simulink subsystem "Genset"  (R2022a)
settings: Solver=VariableStepAuto  StartTime=0.0  StopTime=10  RelTol=1e-3
model mask{Engine=Stellantis 3.0L, Generator=Yasa P400RHC x2}
  mask prompts: Engine "Select an Engine"; Generator "Select a Generator"
undefined symbols (not defined in the file or in its folder): Eng_BSFC_Map, Eng_Const_Power, Eng_Peak_RPM, Eng_Peak_Torque, Eng_RPM_Big, Eng_RPM_Map, Eng_Torque_Big, Eng_Torque_Map, Eng_Torque_Matrix, Gen_Max_Torque, Gen_Max_Torque_line, Gen_RPM_Map, Gen_Torque_Map, P_const_FCA, T_mat_FCA, w_CE_row
libraries: visionstatistics x4, simulink x2, slpidlib x1
settings Model: DefaultTestHarness=Genset_Harness3  Creator=kashyab  LastModifiedBy=kashyab

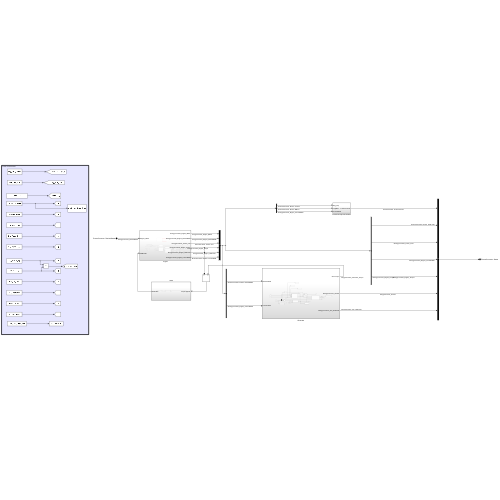
[thumbnail: Simulink's stored preview of the top-level diagram]
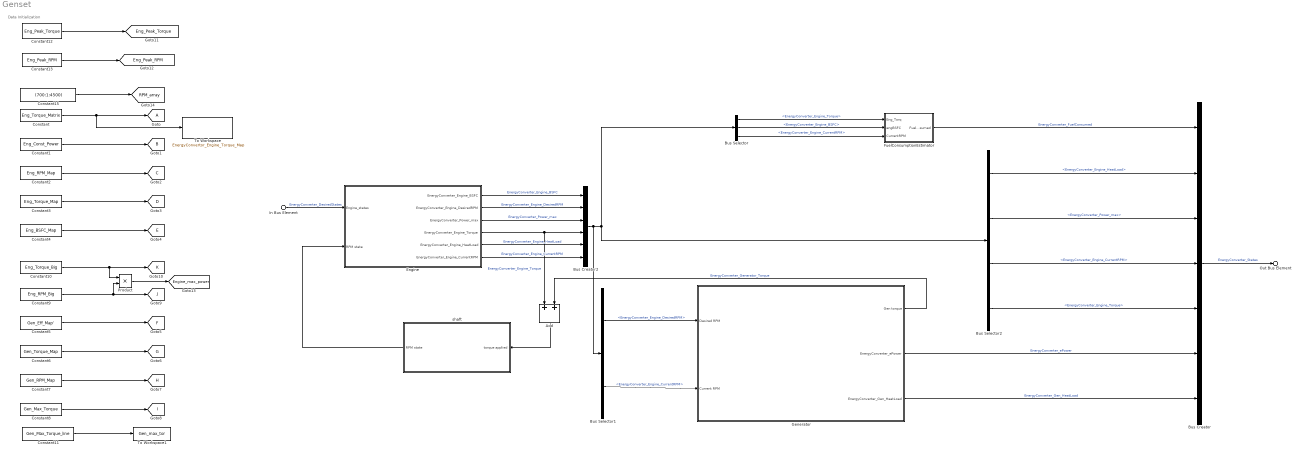
== system Genset ==
  note: Data Initialization
  In Bus Element : Inport  PortName=EnergyConverter_DesiredStates
  Add : Sum
  Bus Creator : BusCreator  Inputs=7
  Bus Creator2 : BusCreator  Inputs=6
  Bus Selector : BusSelector  OutputSignals=EnergyConverter_Engine_Torque,EnergyConverter_Engine_BSFC,EnergyConverter_Engine_CurrentRPM
  Bus Selector1 : BusSelector  OutputSignals=EnergyConverter_Engine_DesiredRPM,EnergyConverter_Engine_CurrentRPM
  Bus Selector2 : BusSelector  OutputSignals=EnergyConverter_Engine_HeatLoad,EnergyConverter_Power_max,EnergyConverter_Engine_CurrentRPM,EnergyConverter_Engine_Torque
  Constant : Constant  Value=Eng_Torque_Matrix
  Constant1 : Constant  Value=Eng_Const_Power
  Constant10 : Constant  Value=Eng_Torque_Big
  Constant11 : Constant  Value=Gen_Max_Torque_line
  Constant12 : Constant  Value=Eng_Peak_Torque
  Constant13 : Constant  Value=Eng_Peak_RPM
  Constant15 : Constant  Value=(700:1:4500)
  Constant2 : Constant  Value=Eng_RPM_Map
  Constant3 : Constant  Value=Eng_Torque_Map
  Constant4 : Constant  Value=Eng_BSFC_Map
  Constant5 : Constant  Value=Gen_Eff_Map'
  Constant6 : Constant  Value=Gen_Torque_Map
  Constant7 : Constant  Value=Gen_RPM_Map
  Constant8 : Constant  Value=Gen_Max_Torque
  Constant9 : Constant  Value=Eng_RPM_Big
  Engine : Subsystem
  FuelConsumptionEstimator : Subsystem
  Generator : Subsystem
  Goto : Goto  TagVisibility=global
  Product : Product
  To Workspace : ToWorkspace  VariableName=EnergyConvertor_Engine_Torque_Map  SampleTime=-1
      settings: Save2DSignal=2-D array (concatenate along first dimension)
  To Workspace1 : ToWorkspace  VariableName=Gen_max_tor  SaveFormat=Timeseries  SampleTime=-1
  shaft : Subsystem
  Out Bus Element : Outport  PortName=EnergyConverter_States
  tag scope: B=global, C=global, D=global, E=global, Eng_Peak_RPM=global, Eng_Peak_Torque=global, Engine_max_power=global, F=global, G=global, H=global, I=global, J=global, K=global, RPM_array=global
  wires:
  Generator/2(EnergyConverter_ePower) -> Bus Creator/6  "EnergyConverter_ePower"
  Bus Creator/1 -> Out Bus Element/1  "EnergyConverter_States"
  Constant8/1 -> [I]
  Constant7/1 -> [H]
  Constant6/1 -> [G]
  Constant5/1 -> [F]
  Constant4/1 -> [E]
  Constant3/1 -> [D]
  Constant2/1 -> [C]
  Constant1/1 -> [B]
  Constant/1 -> Goto/1, To Workspace/1
  Add/1 -> shaft/1("torque applied ")
  shaft/1(RPM state) -> Engine/2(RPM state)
  Generator/1("Gen torque ") -> Add/2  "EnergyConverter_Generator_Torque"
  Bus Selector2/3 -> Bus Creator/4  "<EnergyConverter_Engine_CurrentRPM>"
  Bus Selector2/2 -> Bus Creator/3  "<EnergyConverter_Power_max>"
  Constant9/1 -> [J], Product/2
  Generator/3(EnergyConverter_Gen_HeatLoad) -> Bus Creator/7  "EnergyConverter_Gen_HeatLoad"
  FuelConsumptionEstimator/1(FuelConsumed) -> Bus Creator/1  "EnergyConverter_FuelConsumed"
  Bus Selector2/1 -> Bus Creator/2  "<EnergyConverter_Engine_HeatLoad>"
  Constant11/1 -> To Workspace1/1
  Constant12/1 -> [Eng_Peak_Torque]
  Constant13/1 -> [Eng_Peak_RPM]
  Constant10/1 -> Product/1, [K]
  Product/1 -> [Engine_max_power]
  Constant15/1 -> [RPM_array]
  Engine/1(EnergyConverter_Engine_BSFC) -> Bus Creator2/1  "EnergyConverter_Engine_BSFC"
  Engine/2(EnergyConverter_Engine_DesiredRPM) -> Bus Creator2/2  "EnergyConverter_Engine_DesiredRPM"
  Engine/3(EnergyConverter_Power_max) -> Bus Creator2/3  "EnergyConverter_Power_max"
  Engine/4(" EnergyConverter_Engine_Torque") -> Bus Creator2/4, Add/1  "EnergyConverter_Engine_Torque"
  Engine/5(EnergyConverter_Engine_HeatLoad) -> Bus Creator2/5  "EnergyConverter_Engine_HeatLoad"
  Engine/6(EnergyConverter_Engine_CurrentRPM) -> Bus Creator2/6  "EnergyConverter_Engine_CurrentRPM"
  Bus Creator2/1 -> Bus Selector/1, Bus Selector2/1, Bus Selector1/1
  Bus Selector/1 -> FuelConsumptionEstimator/1(Eng_Torq)  "<EnergyConverter_Engine_Torque>"
  Bus Selector/2 -> FuelConsumptionEstimator/2(engBSFC)  "<EnergyConverter_Engine_BSFC>"
  Bus Selector/3 -> FuelConsumptionEstimator/3(CurrentRPM)  "<EnergyConverter_Engine_CurrentRPM>"
  Bus Selector1/1 -> Generator/1(Desired RPM)  "<EnergyConverter_Engine_DesiredRPM>"
  Bus Selector1/2 -> Generator/2(Current RPM)  "<EnergyConverter_Engine_CurrentRPM>"
  In Bus Element/1 -> Engine/1(Engine_states)  "EnergyConverter_DesiredStates"
  Bus Selector2/4 -> Bus Creator/5  "<EnergyConverter_Engine_Torque>"

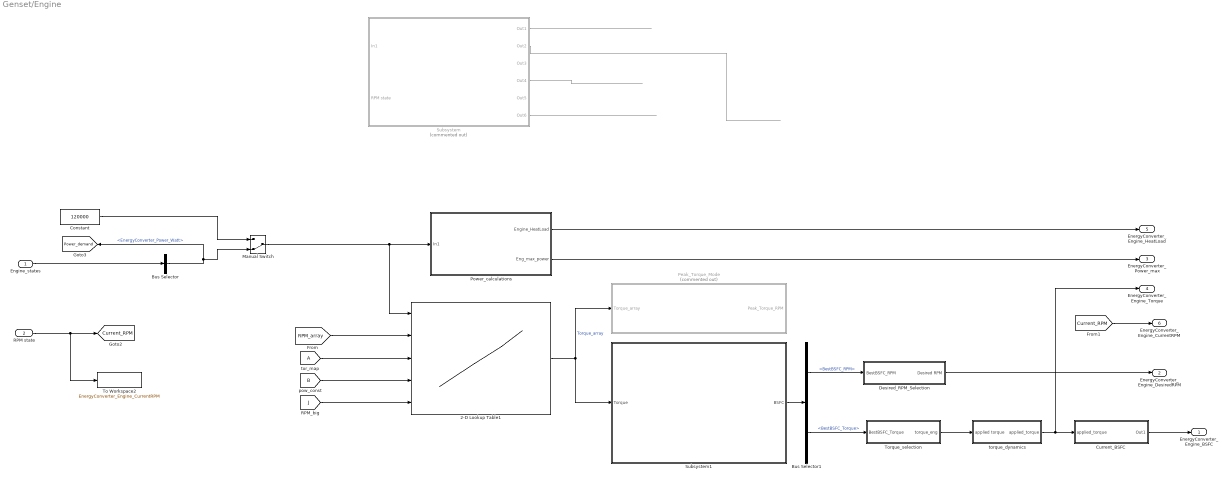
== system Genset/Engine ==
  Engine_states : Inport
  RPM state : Inport  Port=2
  2-D Lookup Table1 : Lookup_n-D  BreakpointsForDimension1Source=Input port  BreakpointsForDimension1=P_const_FCA  BreakpointsForDimension2Source=Input port  BreakpointsForDimension2=w_CE_row  IndexSearchMethod=Linear search  TableSource=Input port  Table=T_mat_FCA  ExtrapMethod=Clip  UseLastTableValue=on  InternalRulePriority=Speed  RndMeth=Simplest
      settings: InputPortMap=u0,u1,p221,p5,p7
  Bus Selector : BusSelector  OutputSignals=EnergyConverter_Power_Watt
  Bus Selector1 : BusSelector  OutputSignals=BestBSFC_RPM,BestBSFC_Torque
  Constant : Constant  Value=120000
  Current_BSFC : Subsystem
  Desired_RPM_Selection : Subsystem
  Manual Switch : ManualSwitch  CurrentSetting=0
  Peak_Torque_Mode : Subsystem  Commented=on
  Power_calculations : Subsystem
  Subsystem : Subsystem  Commented=on
  Subsystem1 : Subsystem
  To Workspace2 : ToWorkspace  VariableName=EnergyConverter_Engine_CurrentRPM  SampleTime=-1
      settings: Save2DSignal=2-D array (concatenate along first dimension)
  Torque_selection : Subsystem
  tor_map : From  TagVisibility=global
  torque_dynamics : Subsystem
  EnergyConverter_Engine_BSFC : Outport
  EnergyConverter_Engine_DesiredRPM : Outport  Port=2
  EnergyConverter_Power_max : Outport  Port=3
  " EnergyConverter_Engine_Torque" : Outport  Port=4
  EnergyConverter_Engine_HeatLoad : Outport  Port=5
  EnergyConverter_Engine_CurrentRPM : Outport  Port=6
  tag scope: Current_RPM=global, Power_demand=global
  wires:
  [RPM_array] -> 2-D Lookup Table1/2
  2-D Lookup Table1/1 -> Peak_Torque_Mode/1(Torque_array), Subsystem1/1(Torque)  "Torque_array"
  [B] -> 2-D Lookup Table1/4
  [J] -> 2-D Lookup Table1/5
  tor_map/1 -> 2-D Lookup Table1/3
  Subsystem/6(Out6) -> ?
  Subsystem/4(Out4) -> ?
  Subsystem/2(Out2) -> ?
  Subsystem/1(Out1) -> ?
  RPM state/1 -> [Current_RPM], To Workspace2/1
  Manual Switch/1 -> Power_calculations/1(In1), 2-D Lookup Table1/1
  Bus Selector/1 -> Manual Switch/2, [Power_demand]  "<EnergyConverter_Power_Watt>"
  Engine_states/1 -> Bus Selector/1
  Constant/1 -> Manual Switch/1
  Subsystem1/1(BSFC) -> Bus Selector1/1
  Bus Selector1/1 -> Desired_RPM_Selection/1(BestBSFC_RPM)  "<BestBSFC_RPM>"
  Bus Selector1/2 -> Torque_selection/1(BestBSFC_Torque)  "<BestBSFC_Torque>"
  Desired_RPM_Selection/1("Desired RPM ") -> EnergyConverter_Engine_DesiredRPM/1
  Torque_selection/1(torque_eng) -> torque_dynamics/1(applied torque)
  torque_dynamics/1(applied_torque) -> " EnergyConverter_Engine_Torque"/1, Current_BSFC/1(applied_torque)
  Current_BSFC/1(Out1) -> EnergyConverter_Engine_BSFC/1
  Power_calculations/2(Eng_max_power) -> EnergyConverter_Power_max/1
  Power_calculations/1(Engine_HeatLoad) -> EnergyConverter_Engine_HeatLoad/1
  [Current_RPM] -> EnergyConverter_Engine_CurrentRPM/1

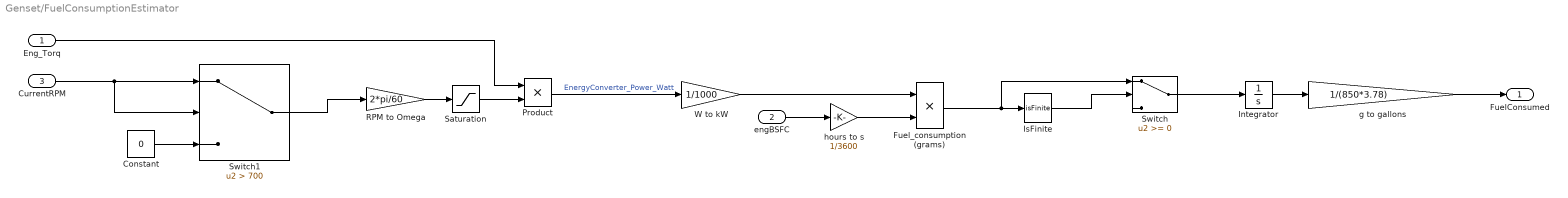
== system Genset/FuelConsumptionEstimator ==
  Eng_Torq : Inport
  engBSFC : Inport  Port=2
  CurrentRPM : Inport  Port=3
  Constant : Constant  Value=0
  Fuel_consumption (grams) : Product
  Integrator : Integrator
  IsFinite : RelationalOperator  Operator=isFinite  OutDataTypeStr=boolean  RndMeth=Simplest  InputSameDT=off
  Product : Product
  RPM to Omega : Gain  Gain=2*pi/60
  Saturation : Saturate  UpperLimit=Inf  LowerLimit=0
  Switch : Switch  SaturateOnIntegerOverflow=off  InputSameDT=off
  Switch1 : Switch  Criteria=u2 > Threshold  Threshold=700  SaturateOnIntegerOverflow=off  InputSameDT=off
  W to kW : Gain  Gain=1/1000
  g to gallons : Gain  Gain=1/(850*3.78)
  hours to s : Gain  Gain=1/3600
  FuelConsumed : Outport
  wires:
  Switch1/1 -> RPM to Omega/1
  Constant/1 -> Switch1/3
  Saturation/1 -> Product/2
  Switch/1 -> Integrator/1
  IsFinite/1 -> Switch/2
  Fuel_consumption (grams)/1 -> IsFinite/1, Switch/1
  Integrator/1 -> g to gallons/1
  engBSFC/1 -> hours to s/1
  Product/1 -> W to kW/1  "EnergyConverter_Power_Watt"
  RPM to Omega/1 -> Saturation/1
  CurrentRPM/1 -> Switch1/1, Switch1/2
  Eng_Torq/1 -> Product/1
  g to gallons/1 -> FuelConsumed/1
  hours to s/1 -> Fuel_consumption (grams)/2
  W to kW/1 -> Fuel_consumption (grams)/1

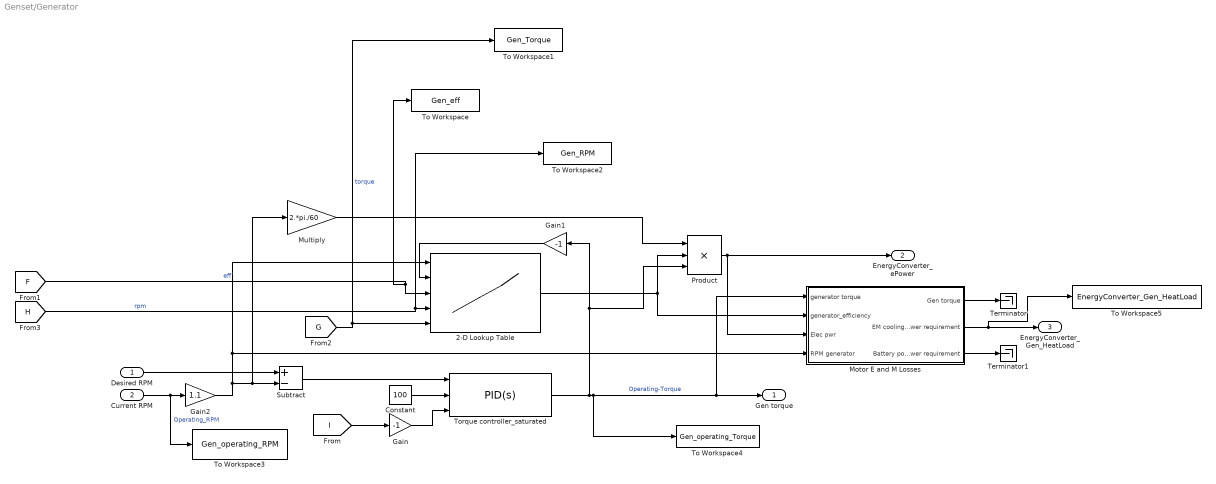
== system Genset/Generator ==
  Desired RPM : Inport
  Current RPM : Inport  Port=2
  2-D Lookup Table : Lookup_n-D  BreakpointsForDimension1Source=Input port  BreakpointsForDimension1=[1:3]  BreakpointsForDimension2Source=Input port  BreakpointsForDimension2=[1:3]  TableSource=Input port  ExtrapMethod=Clip  UseLastTableValue=on  InternalRulePriority=Speed  RndMeth=Simplest
      settings: InputPortMap=u0,u1,p221,p5,p7
  Constant : Constant  Value=100
  Gain : Gain  Gain=-1
  Gain1 : Gain  Gain=-1
  Gain2 : Gain  Gain=1.1
  Motor E and M Losses : Subsystem
  Multiply : Gain  Gain=2.*pi./60
  Product : Product  Inputs=3
  Subtract : Sum  Inputs=+-
  Terminator : Terminator
  Terminator1 : Terminator
  To Workspace : ToWorkspace  VariableName=Gen_eff  SaveFormat=Timeseries  SampleTime=-1
  To Workspace1 : ToWorkspace  VariableName=Gen_Torque  SaveFormat=Timeseries  SampleTime=-1
  To Workspace2 : ToWorkspace  VariableName=Gen_RPM  SaveFormat=Timeseries  SampleTime=-1
  To Workspace3 : ToWorkspace  VariableName=Gen_operating_RPM  SampleTime=-1
      settings: Save2DSignal=2-D array (concatenate along first dimension)
  To Workspace4 : ToWorkspace  VariableName=Gen_operating_Torque  SampleTime=-1
      settings: Save2DSignal=2-D array (concatenate along first dimension)
  To Workspace5 : ToWorkspace  VariableName=EnergyConverter_Gen_HeatLoad  SampleTime=-1
      settings: Save2DSignal=2-D array (concatenate along first dimension)
  Torque controller_saturated : slpidlib/PID Controller  Controller=PID  Form=Parallel  TimeDomain=Continuous-time  UseExternalTs=off  SampleTime=-1  IntegratorMethod=Forward Euler  FilterMethod=Forward Euler  ControllerParametersSource=internal  P=7.5  I=.5  UseKiTs=off  D=0  N=100  UseFilter=on  TunerSelectOption=Transfer Function Based (PID Tuner App)  InitialConditionSource=internal  InitialConditionForIntegrator=0  InitialConditionForFilter=0  DifferentiatorICPrevScaledInput=0  ExternalReset=none  TrackingMode=off  Kt=1  LimitOutput=on  SatLimitsSource=external  UpperSaturationLimit=0  LowerSaturationLimit=-650  LinearizeAsGain=on  AntiWindupMode=none  Kb=1  POutMin=[]  POutMax=[]  IOutMin=[]  IOutMax=[]  DOutMin=[]  DOutMax=[]  NOutMin=[]  NOutMax=[]  SumOutMin=[]  SumOutMax=[]  SaturationOutMin=[]  SaturationOutMax=[]  PParamMin=[]  PParamMax=[]  IParamMin=[]  IParamMax=[]  DParamMin=[]  DParamMax=[]  NParamMin=[]  NParamMax=[]  KbParamMin=[]  KbParamMax=[]  KtParamMin=[]  KtParamMax=[]  KbOutMin=[]  KbOutMax=[]  KtOutMin=[]  KtOutMax=[]  IntegratorOutMin=[]  IntegratorOutMax=[]  FilterOutMin=[]  FilterOutMax=[]  SumI1OutMin=[]  SumI1OutMax=[]  SumI2OutMin=[]  SumI2OutMax=[]  SumI3OutMin=[]  SumI3OutMax=[]  SumI4OutMin=[]  SumI4OutMax=[]  SumDOutMin=[]  SumDOutMax=[]  DifferentiatorOutMin=[]  DifferentiatorOutMax=[]  FilterDiffOutCoefMin=[]  FilterDiffOutCoefMax=[]  ReciprocalOutMin=[]  ReciprocalOutMax=[]  SumDenOutMin=[]  SumDenOutMax=[]  SumNumOutMin=[]  SumNumOutMax=[]  DivideOutMin=[]  DivideOutMax=[]  UdiffTsProdOutMin=[]  UdiffTsProdOutMax=[]  NTsProdOutMin=[]  NTsProdOutMax=[]  UintegralTsProdOutMin=[]  UintegralTsProdOutMax=[]  UngainTsProdOutMin=[]  UngainTsProdOutMax=[]  IntegratorContinuousStateAttributes=''  IntegratorStateMustResolveToSignalObject=off  IntegratorRTWStateStorageClass=Auto  FilterContinuousStateAttributes=''  FilterStateMustResolveToSignalObject=off  FilterRTWStateStorageClass=Auto  ParallelPVariant=InternalParameters  IdealPVariant=Disabled  IVariant=InternalParameters  DVariant=InternalParameters  IntegratorVariant=Continuous  SatVariant=External  AWVariant=Passthrough  PCopyVariant=Disabled  TRVariant=Disabled  FdbkBlocksVariant=Forward  IdealPFdbkVariant=Disabled  SatFdbkVariant=Disabled  DerivativeFilterVariant=ContFilter  NVariant=InternalParameters  NCopyVariant=Disabled  FilterICVariant=InternalICsFilter  IntegratorICVariant=InternalICs  ExternalResetVariant=Disabled  TRSumVariant=Passthrough  SumFdbkVariant=Disabled  SumVariant=Sum_PID  TsampFilterVariant=InternalTs  TsampNgainVariant=Passthrough  TsampIntegralVariant=Passthrough  ExternalSaturationOutDataTypeStr=Inherit: Same as second input  aMode=0
  "Gen torque " : Outport
  EnergyConverter_ePower : Outport  Port=2
  EnergyConverter_Gen_HeatLoad : Outport  Port=3
  wires:
  Gain2/1 -> 2-D Lookup Table/1, Motor E and M Losses/4(RPM generator), Multiply/1, Subtract/2
  Desired RPM/1 -> Subtract/1
  [F] -> 2-D Lookup Table/3, To Workspace/1  "eff"
  Torque controller_saturated/1 -> Motor E and M Losses/1(generator torque), "Gen torque "/1, To Workspace4/1, Gain1/1, Product/3  "Operating-Torque"
  Subtract/1 -> Torque controller_saturated/1
  Current RPM/1 -> To Workspace3/1, Gain2/1  "Operating_RPM"
  2-D Lookup Table/1 -> Product/2, Motor E and M Losses/2(generator_efficiency)
  Constant/1 -> Torque controller_saturated/2
  [I] -> Gain/1
  Gain/1 -> Torque controller_saturated/3
  Multiply/1 -> Product/1
  Product/1 -> Motor E and M Losses/3(Elec pwr), EnergyConverter_ePower/1
  [H] -> To Workspace2/1, 2-D Lookup Table/4  "rpm"
  [G] -> 2-D Lookup Table/5, To Workspace1/1  "torque"
  Gain1/1 -> 2-D Lookup Table/2
  Motor E and M Losses/3(Battery power requirement) -> Terminator1/1
  Motor E and M Losses/1(Gen torque) -> Terminator/1
  Motor E and M Losses/2(EM cooling power requirement) -> To Workspace5/1, EnergyConverter_Gen_HeatLoad/1

== system Genset/shaft ==
  "torque applied " : Inport
  Gain : Gain  Gain=10
  Integrator : Integrator  InitialCondition=1
  RPM state : Outport
  wires:
  Gain/1 -> Integrator/1
  Integrator/1 -> RPM state/1
  "torque applied "/1 -> Gain/1

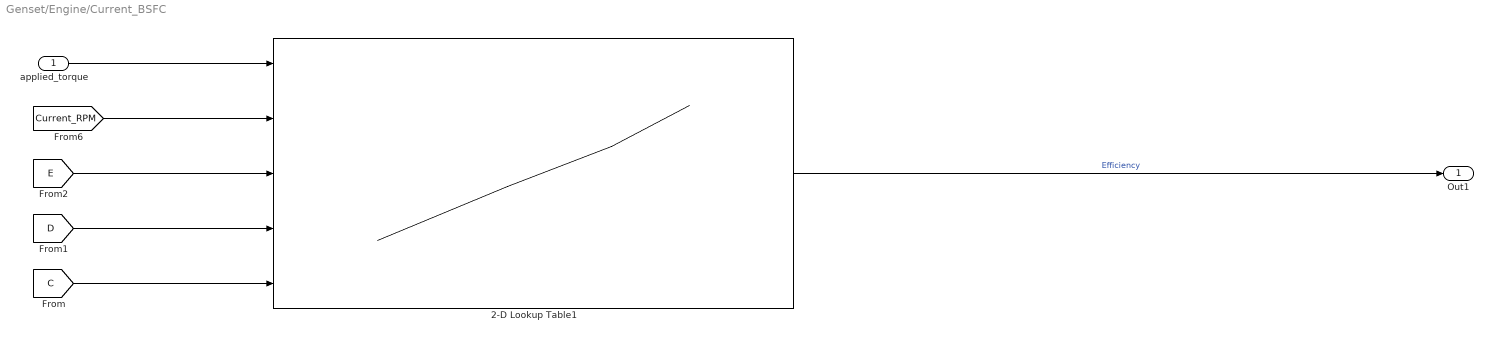
== system Genset/Engine/Current_BSFC ==
  applied_torque : Inport
  2-D Lookup Table1 : Lookup_n-D  BreakpointsForDimension1Source=Input port  BreakpointsForDimension1=[1:3]  BreakpointsForDimension2Source=Input port  BreakpointsForDimension2=[1:3]  TableSource=Input port  ExtrapMethod=Clip  UseLastTableValue=on  InternalRulePriority=Speed  RndMeth=Simplest
      settings: InputPortMap=u0,u1,p221,p5,p7
  Out1 : Outport
  wires:
  [Current_RPM] -> 2-D Lookup Table1/2
  2-D Lookup Table1/1 -> Out1/1  "Efficiency"
  applied_torque/1 -> 2-D Lookup Table1/1
  [D] -> 2-D Lookup Table1/4
  [E] -> 2-D Lookup Table1/3
  [C] -> 2-D Lookup Table1/5

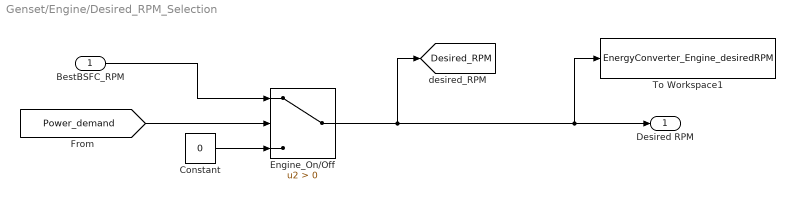
== system Genset/Engine/Desired_RPM_Selection ==
  BestBSFC_RPM : Inport
  Constant : Constant  Value=0
  Engine_On/Off : Switch  Criteria=u2 > Threshold  SaturateOnIntegerOverflow=off  InputSameDT=off
  To Workspace1 : ToWorkspace  VariableName=EnergyConverter_Engine_desiredRPM  SampleTime=-1
      settings: Save2DSignal=2-D array (concatenate along first dimension)
  "Desired RPM " : Outport
  tag scope: Desired_RPM=global
  wires:
  Engine_On/Off/1 -> "Desired RPM "/1, To Workspace1/1, [Desired_RPM]
  [Power_demand] -> Engine_On/Off/2
  Constant/1 -> Engine_On/Off/3
  BestBSFC_RPM/1 -> Engine_On/Off/1

== system Genset/Engine/Peak_Torque_Mode ==
  Torque_array : Inport
  Max RPM : MultiPortSwitch  DataPortOrder=Zero-based contiguous  Inputs=1  zeroidx=on  SaturateOnIntegerOverflow=off  InputSameDT=off
  Max Torque : visionstatistics/2-D Maximum  fcn=Index  reset=None  indexBase=One  operateOver=Entire input  Dimension=1  colComp=on  operation=maximum  accumLastDataTypeStr=Inherit: Same as product output  roiEnable=off  roiType=Rectangles  roiPortion=Entire ROI  roiOutput=Individual statistics for each ROI  roiFlag=off  roundingMode=Floor  overflowMode=off  accumDataTypeStr=Inherit: Same as product output
      settings: SourceProductBaseCode=VP
  Peak_Torque_RPM : Outport
  wires:
  Torque_array/1 -> Max Torque/1
  [RPM_array] -> Max RPM/2
  Max Torque/1 -> Max RPM/1
  Max RPM/1 -> Peak_Torque_RPM/1

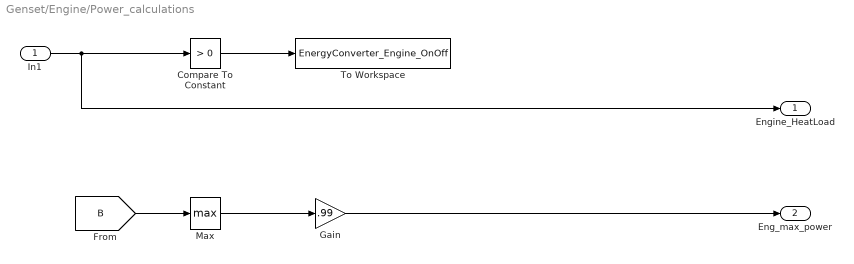
== system Genset/Engine/Power_calculations ==
  In1 : Inport
  Compare To Constant : simulink/Logic and Bit Operations/Compare To Constant  relop=>  const=0  OutDataTypeStr=boolean
  Gain : Gain  Gain=.99
  Max : MinMax  Function=max
  To Workspace : ToWorkspace  VariableName=EnergyConverter_Engine_OnOff  SampleTime=-1
      settings: Save2DSignal=2-D array (concatenate along first dimension)
  Engine_HeatLoad : Outport
  Eng_max_power : Outport  Port=2
  wires:
  In1/1 -> Engine_HeatLoad/1, Compare To Constant/1
  Compare To Constant/1 -> To Workspace/1
  [B] -> Max/1
  Max/1 -> Gain/1
  Gain/1 -> Eng_max_power/1

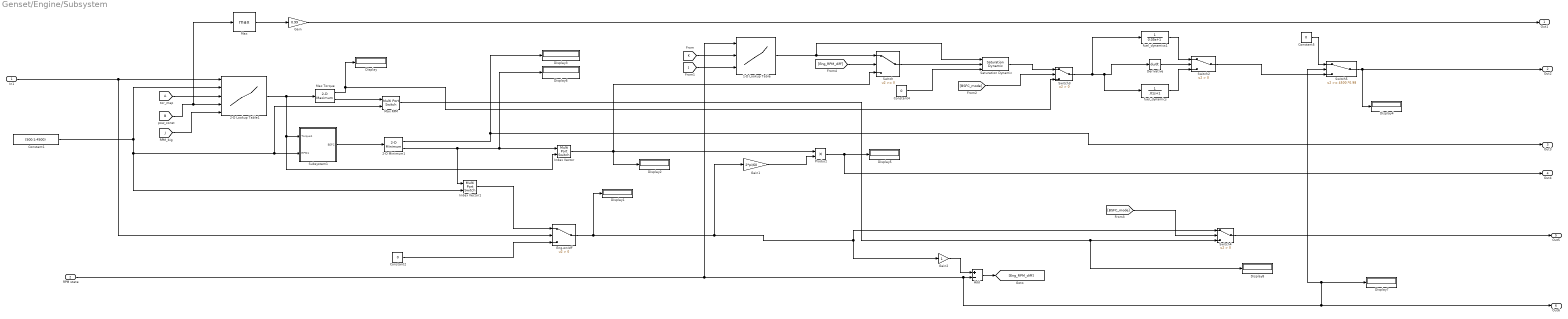
== system Genset/Engine/Subsystem ==
  In1 : Inport
  RPM state : Inport  Port=2
  1-D Lookup Table : Lookup_n-D  NumberOfTableDimensions=1  BreakpointsForDimension1Source=Input port  BreakpointsForDimension1=[-5:5]  TableSource=Input port  Table=tanh([-5:5])  ExtrapMethod=Clip  UseLastTableValue=on  InternalRulePriority=Speed  RndMeth=Simplest
      settings: InputPortMap=u0,p221,p5
  2-D Lookup Table1 : Lookup_n-D  BreakpointsForDimension1Source=Input port  BreakpointsForDimension1=P_const_FCA  BreakpointsForDimension2Source=Input port  BreakpointsForDimension2=w_CE_row  IndexSearchMethod=Linear search  TableSource=Input port  Table=T_mat_FCA  ExtrapMethod=Clip  UseLastTableValue=on  InternalRulePriority=Speed  RndMeth=Simplest
      settings: InputPortMap=u0,u1,p221,p5,p7
  2-D Minimum1 : visionstatistics/2-D Minimum  fcn=Value and Index  reset=None  indexBase=One  operateOver=Entire input  Dimension=1  colComp=on  operation=minimum  accumLastDataTypeStr=Inherit: Same as product output  roiEnable=off  roiType=Rectangles  roiPortion=Entire ROI  roiOutput=Individual statistics for each ROI  roiFlag=off  roundingMode=Floor  overflowMode=off  accumDataTypeStr=Inherit: Same as product output
      settings: SourceProductBaseCode=VP
  Add : Sum  Inputs=+-
  Constant1 : Constant  Value=(500:1:4500)
  Constant2 : Constant  Value=0
  Constant4 : Constant  Value=0
  Constant5 : Constant  Value=0
  Derivative : Derivative
  Display{,1..8} (9 alike) : Display
      Display3 settings: Decimation=4
      Display6 settings: Decimation=4
  Eng-on/off : Switch  Criteria=u2 > Threshold  SaturateOnIntegerOverflow=off  InputSameDT=off
  Gain : Gain  Gain=0.99
  Gain1 : Gain  Gain=2*pi/60
  Gain2 : Gain
  Index Vector : MultiPortSwitch  Inputs=1  SaturateOnIntegerOverflow=off  InputSameDT=off
  Index Vector1 : MultiPortSwitch  Inputs=1  SaturateOnIntegerOverflow=off  InputSameDT=off
  Max : MinMax  Function=max
  Max RPM : MultiPortSwitch  DataPortOrder=Zero-based contiguous  Inputs=1  zeroidx=on  SaturateOnIntegerOverflow=off  InputSameDT=off
  Max Torque : visionstatistics/2-D Maximum  fcn=Value and Index  reset=None  indexBase=One  operateOver=Entire input  Dimension=1  colComp=on  operation=maximum  accumLastDataTypeStr=Inherit: Same as product output  roiEnable=off  roiType=Rectangles  roiPortion=Entire ROI  roiOutput=Individual statistics for each ROI  roiFlag=off  roundingMode=Floor  overflowMode=off  accumDataTypeStr=Inherit: Same as product output
      settings: SourceProductBaseCode=VP
  Product : Product
  Saturation Dynamic : simulink/Discontinuities/Saturation Dynamic  OutMin=[]  OutMax=[]  OutDataTypeStr=Inherit: Same as second input  OutDataType=fixdt(1, 16)  OutScaling=2^-10  DoSatur=off
  Subsystem1 : Subsystem
  Switch : Switch  SaturateOnIntegerOverflow=off  InputSameDT=off
  Switch2 : Switch  Criteria=u2 > Threshold  SaturateOnIntegerOverflow=off  InputSameDT=off
  Switch3 : Switch  Criteria=u2 > Threshold  SaturateOnIntegerOverflow=off  InputSameDT=off
  Switch4 : Switch  Criteria=u2 > Threshold  SaturateOnIntegerOverflow=off  InputSameDT=off
  Switch5 : Switch  Threshold=4500.*0.98  SaturateOnIntegerOverflow=off  InputSameDT=off
  fuel_dynamics : TransferFcn  Denominator=[.01 1]
  fuel_dynamics1 : TransferFcn  Denominator=[0.05 1]
  tor_map : From  TagVisibility=global
  Out1 : Outport
  Out2 : Outport  Port=2
  Out3 : Outport  Port=3
  Out4 : Outport  Port=4
  Out5 : Outport  Port=5
  Out6 : Outport  Port=6
  wires:
  fuel_dynamics/1 -> Switch2/3
  fuel_dynamics1/1 -> Switch2/1
  Derivative/1 -> Switch2/2
  Switch3/1 -> Derivative/1, fuel_dynamics/1, fuel_dynamics1/1
  Constant4/1 -> Saturation Dynamic/3
  Max Torque/1 -> Switch3/3, Display/1
  In1/1 -> 2-D Lookup Table1/1, Eng-on/off/2
  1-D Lookup Table/1 -> Switch/1, Saturation Dynamic/1
  Add/1 -> [Eng_RPM_diff]
  Max/1 -> Gain/1
  tor_map/1 -> 2-D Lookup Table1/3
  RPM state/1 -> 1-D Lookup Table/1, Add/2, Switch5/2, Display7/1, Out6/1
  Switch4/1 -> Out5/1
  Gain/1 -> Out1/1
  [Eng_RPM_diff] -> Switch/2
  [J] -> 2-D Lookup Table1/5
  Max Torque/2 -> Max RPM/1
  [K] -> 1-D Lookup Table/2
  Gain2/1 -> Add/1
  Constant2/1 -> Eng-on/off/3
  Constant1/1 -> 2-D Lookup Table1/2, Index Vector1/2, Subsystem1/2(RPM1), Max RPM/2
  Index Vector/1 -> Switch/3, Display2/1, Product/1
  [BSFC_mode] -> Switch4/2
  Max RPM/1 -> Switch4/3, Display8/1
  2-D Lookup Table1/1 -> Index Vector/2, Subsystem1/1(Torque1), Max Torque/1
  Saturation Dynamic/1 -> Switch3/1
  [J] -> 1-D Lookup Table/3
  [BSFC_mode] -> Switch3/2
  Index Vector1/1 -> Eng-on/off/1
  2-D Minimum1/2 -> Display6/1, Index Vector/1, Index Vector1/1
  Subsystem1/1(BSFC) -> 2-D Minimum1/1
  Switch5/1 -> Display4/1, Out2/1
  Switch2/1 -> Switch5/3
  Constant5/1 -> Switch5/1
  2-D Minimum1/1 -> Display3/1, Out3/1
  Product/1 -> Display5/1, Out4/1
  [B] -> Max/1, 2-D Lookup Table1/4
  Switch/1 -> Saturation Dynamic/2
  Eng-on/off/1 -> Display1/1, Gain1/1, Gain2/1, Switch4/1
  Gain1/1 -> Product/2

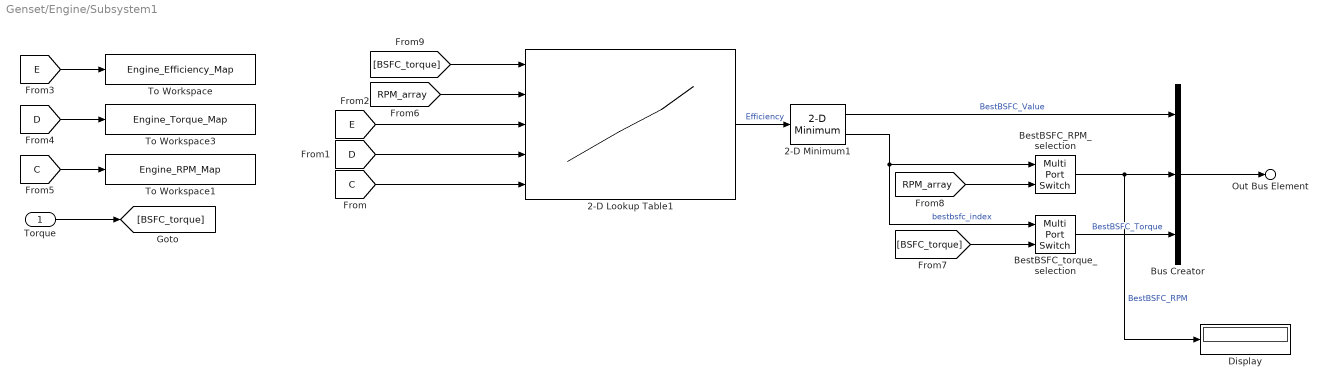
== system Genset/Engine/Subsystem1 ==
  Torque : Inport
  2-D Lookup Table1 : Lookup_n-D  BreakpointsForDimension1Source=Input port  BreakpointsForDimension1=[1:3]  BreakpointsForDimension2Source=Input port  BreakpointsForDimension2=[1:3]  TableSource=Input port  ExtrapMethod=Clip  UseLastTableValue=on  InternalRulePriority=Speed  RndMeth=Simplest
      settings: InputPortMap=u0,u1,p221,p5,p7
  2-D Minimum1 : visionstatistics/2-D Minimum  fcn=Value and Index  reset=None  indexBase=One  operateOver=Entire input  Dimension=1  colComp=on  operation=minimum  accumLastDataTypeStr=Inherit: Same as product output  roiEnable=off  roiType=Rectangles  roiPortion=Entire ROI  roiOutput=Individual statistics for each ROI  roiFlag=off  roundingMode=Floor  overflowMode=off  accumDataTypeStr=Inherit: Same as product output
      settings: SourceProductBaseCode=VP
  BestBSFC_RPM_selection : MultiPortSwitch  Inputs=1  SaturateOnIntegerOverflow=off  InputSameDT=off
  BestBSFC_torque_selection : MultiPortSwitch  Inputs=1  SaturateOnIntegerOverflow=off  InputSameDT=off
  Bus Creator : BusCreator  Inputs=3
  Display : Display
  To Workspace : ToWorkspace  VariableName=Engine_Efficiency_Map  SampleTime=-1
      settings: Save2DSignal=2-D array (concatenate along first dimension)
  To Workspace1 : ToWorkspace  VariableName=Engine_RPM_Map  SampleTime=-1
      settings: Save2DSignal=2-D array (concatenate along first dimension)
  To Workspace3 : ToWorkspace  VariableName=Engine_Torque_Map  SampleTime=-1
      settings: Save2DSignal=2-D array (concatenate along first dimension)
  Out Bus Element : Outport  PortName=BSFC
  wires:
  [BSFC_torque] -> 2-D Lookup Table1/1
  BestBSFC_torque_selection/1 -> Bus Creator/3  "BestBSFC_Torque"
  BestBSFC_RPM_selection/1 -> Bus Creator/2, Display/1  "BestBSFC_RPM"
  [RPM_array] -> BestBSFC_RPM_selection/2
  [BSFC_torque] -> BestBSFC_torque_selection/2
  Bus Creator/1 -> Out Bus Element/1
  2-D Minimum1/2 -> BestBSFC_RPM_selection/1, BestBSFC_torque_selection/1  "bestbsfc_index"
  2-D Minimum1/1 -> Bus Creator/1  "BestBSFC_Value"
  [C] -> To Workspace1/1
  [D] -> To Workspace3/1
  [E] -> To Workspace/1
  [C] -> 2-D Lookup Table1/5
  [RPM_array] -> 2-D Lookup Table1/2
  Torque/1 -> [BSFC_torque]
  2-D Lookup Table1/1 -> 2-D Minimum1/1  "Efficiency"
  [E] -> 2-D Lookup Table1/3
  [D] -> 2-D Lookup Table1/4

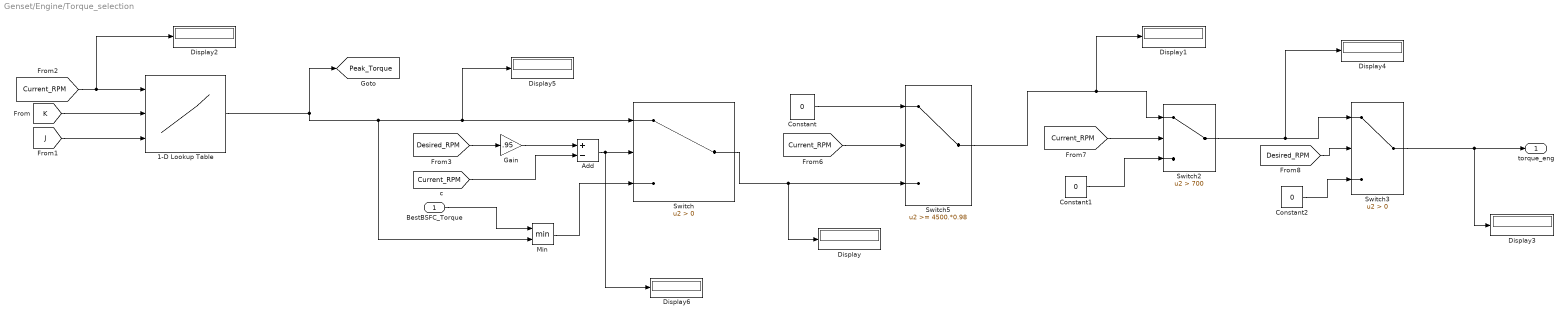
== system Genset/Engine/Torque_selection ==
  BestBSFC_Torque : Inport
  1-D Lookup Table : Lookup_n-D  NumberOfTableDimensions=1  BreakpointsForDimension1Source=Input port  BreakpointsForDimension1=[-5:5]  TableSource=Input port  Table=tanh([-5:5])  ExtrapMethod=Clip  UseLastTableValue=on  InternalRulePriority=Speed  RndMeth=Simplest
      settings: InputPortMap=u0,p221,p5
  Add : Sum  Inputs=+-
  Constant : Constant  Value=0
  Constant1 : Constant  Value=0
  Constant2 : Constant  Value=0
  Display{,1..6} (7 alike) : Display
  Gain : Gain  Gain=.95
  Min : MinMax  Inputs=2
  Switch : Switch  Criteria=u2 > Threshold  SaturateOnIntegerOverflow=off  InputSameDT=off
  Switch2 : Switch  Criteria=u2 > Threshold  Threshold=700  SaturateOnIntegerOverflow=off  InputSameDT=off
  Switch3 : Switch  Criteria=u2 > Threshold  SaturateOnIntegerOverflow=off  InputSameDT=off
  Switch5 : Switch  Threshold=4500.*0.98  SaturateOnIntegerOverflow=off  InputSameDT=off
  torque_eng : Outport
  tag scope: Peak_Torque=global
  wires:
  Min/1 -> Switch/3
  BestBSFC_Torque/1 -> Min/1
  Constant2/1 -> Switch3/3
  Switch3/1 -> torque_eng/1, Display3/1
  [Desired_RPM] -> Switch3/2
  Switch2/1 -> Switch3/1, Display4/1
  Switch5/1 -> Switch2/1, Display1/1
  Constant1/1 -> Switch2/3
  [Current_RPM] -> Switch2/2
  1-D Lookup Table/1 -> [Peak_Torque], Display5/1, Switch/1, Min/2
  [J] -> 1-D Lookup Table/3
  [Current_RPM] -> 1-D Lookup Table/1, Display2/1
  [K] -> 1-D Lookup Table/2
  [Desired_RPM] -> Gain/1
  [Current_RPM] -> Add/2
  Gain/1 -> Add/1
  Add/1 -> Switch/2, Display6/1
  [Current_RPM] -> Switch5/2
  Constant/1 -> Switch5/1
  Switch/1 -> Switch5/3, Display/1

== system Genset/Engine/torque_dynamics ==
  applied torque : Inport
  Derivative : Derivative
  Switch2 : Switch  Criteria=u2 > Threshold  SaturateOnIntegerOverflow=off  InputSameDT=off
  fuel_dynamics : TransferFcn  Denominator=[.01 1]
  fuel_dynamics1 : TransferFcn  Denominator=[0.05 1]
  applied_torque : Outport
  wires:
  Switch2/1 -> applied_torque/1
  applied torque/1 -> Derivative/1, fuel_dynamics/1, fuel_dynamics1/1
  fuel_dynamics1/1 -> Switch2/1
  fuel_dynamics/1 -> Switch2/3
  Derivative/1 -> Switch2/2

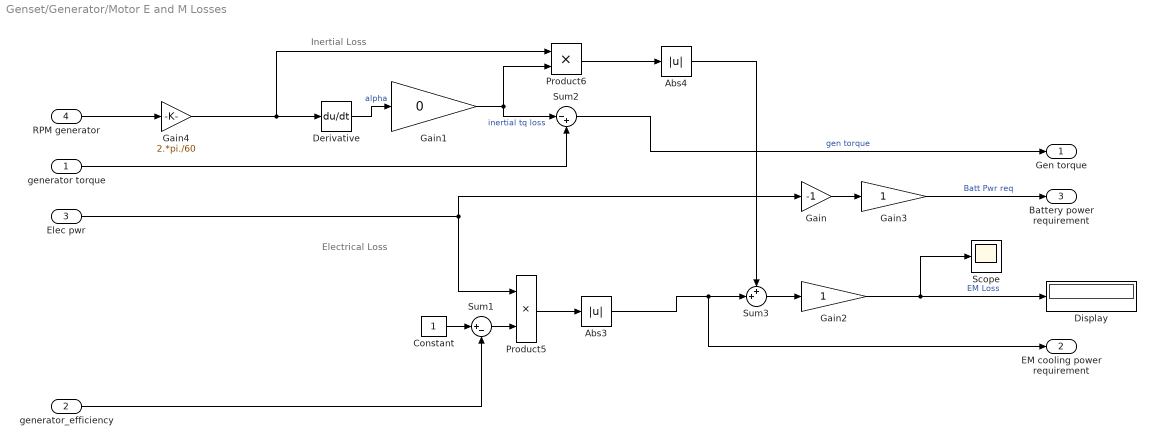
== system Genset/Generator/Motor E and M Losses ==
  note: Inertial Loss
  note: Electrical Loss
  generator torque : Inport
  generator_efficiency : Inport  Port=2
  Elec pwr : Inport  Port=3
  RPM generator : Inport  Port=4
  Abs3 : Abs  SaturateOnIntegerOverflow=off
  Abs4 : Abs  ZeroCross=off  SaturateOnIntegerOverflow=off
  Constant : Constant
  Derivative : Derivative
  Display : Display
  Gain : Gain  Gain=-1
  Gain1 : Gain  Gain=0
  Gain2 : Gain
  Gain3 : Gain
  Gain4 : Gain  Gain=2.*pi./60
  Product5 : Product
  Product6 : Product
  Scope : Scope
  Sum1 : Sum  Inputs=|+-
  Sum2 : Sum  Inputs=|-+
  Sum3 : Sum  Inputs=++|
  Gen torque : Outport
  EM cooling power requirement : Outport  Port=2
  Battery power requirement : Outport  Port=3
  wires:
  Gain4/1 -> Derivative/1, Product6/1
  Gain3/1 -> Battery power requirement/1  "Batt Pwr req"
  Gain/1 -> Gain3/1
  generator_efficiency/1 -> Sum1/2
  Sum2/1 -> Gen torque/1  "gen torque"
  Derivative/1 -> Gain1/1  "alpha"
  Elec pwr/1 -> Product5/1, Gain/1
  Product6/1 -> Abs4/1
  Constant/1 -> Sum1/1
  Abs4/1 -> Sum3/1
  Gain1/1 -> Sum2/1, Product6/2  "inertial tq loss"
  Product5/1 -> Abs3/1
  Gain2/1 -> Scope/1, Display/1  "EM Loss"
  Sum1/1 -> Product5/2
  Sum3/1 -> Gain2/1
  Abs3/1 -> Sum3/2, EM cooling power requirement/1
  RPM generator/1 -> Gain4/1
  generator torque/1 -> Sum2/2

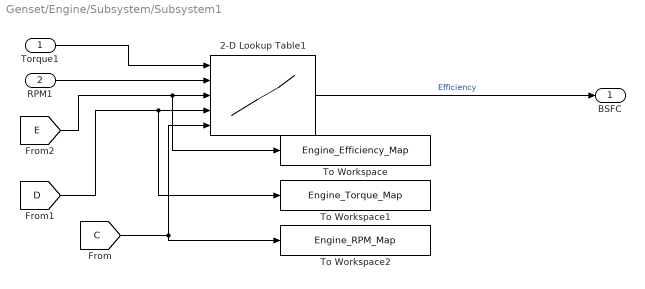
== system Genset/Engine/Subsystem/Subsystem1 ==
  Torque1 : Inport
  RPM1 : Inport  Port=2
  2-D Lookup Table1 : Lookup_n-D  BreakpointsForDimension1Source=Input port  BreakpointsForDimension1=[1:3]  BreakpointsForDimension2Source=Input port  BreakpointsForDimension2=[1:3]  TableSource=Input port  ExtrapMethod=Clip  UseLastTableValue=on  InternalRulePriority=Speed  RndMeth=Simplest
      settings: InputPortMap=u0,u1,p221,p5,p7
  To Workspace : ToWorkspace  VariableName=Engine_Efficiency_Map  SampleTime=-1
      settings: Save2DSignal=2-D array (concatenate along first dimension)
  To Workspace1 : ToWorkspace  VariableName=Engine_Torque_Map  SampleTime=-1
      settings: Save2DSignal=2-D array (concatenate along first dimension)
  To Workspace2 : ToWorkspace  VariableName=Engine_RPM_Map  SampleTime=-1
      settings: Save2DSignal=2-D array (concatenate along first dimension)
  BSFC : Outport
  wires:
  [C] -> To Workspace2/1, 2-D Lookup Table1/5
  RPM1/1 -> 2-D Lookup Table1/2
  Torque1/1 -> 2-D Lookup Table1/1
  2-D Lookup Table1/1 -> BSFC/1  "Efficiency"
  [E] -> 2-D Lookup Table1/3, To Workspace/1
  [D] -> 2-D Lookup Table1/4, To Workspace1/1
